simulink model "engv2_Simscape_test_no_graphs"  (R2016a)
settings: Solver=ode23t  StartTime=0.0  StopTime=5790*3  MaxStep=0.1  RelTol=1e-6
libraries: fl_lib x35, nesl_utility x35, elec_lib x10, simulink x2
settings Model: Creator=Bruno  LastModifiedBy=Bruno Eiterer
settings SolverCC: MaxConsecutiveZCs=10000  ZeroCrossAlgorithm=Adaptive  AlgebraicLoopSolver=LineSearch  SolverResetMethod=Robust

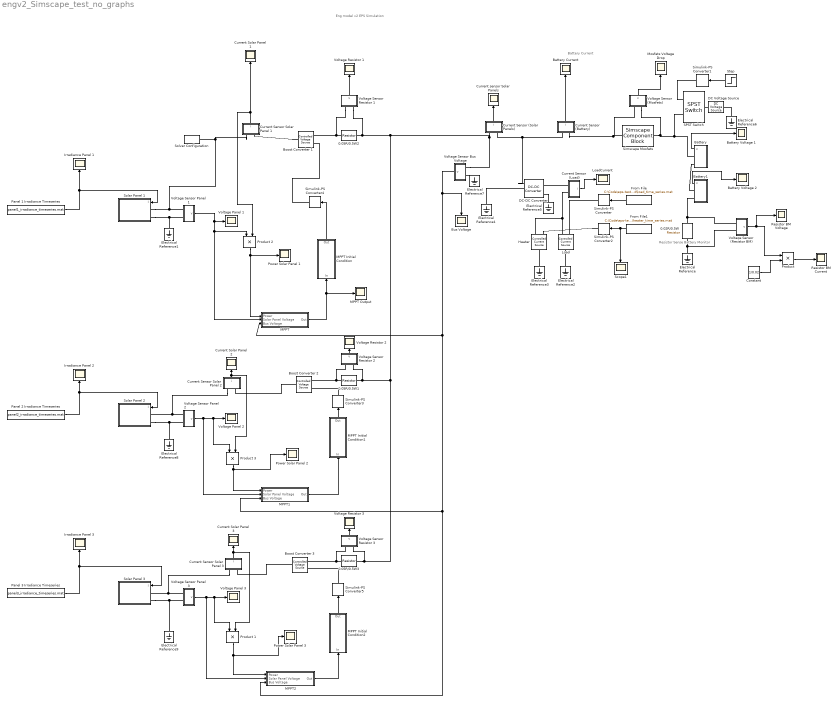
== system engv2_Simscape_test_no_graphs ==
  note: Battery Current
  note: Resistor Sense
      | Battery Monitor
  note: Eng model v2 EPS Simulation
  " Battery" : Subsystem
      settings: CopyFcn=set_param(gcb,'LinkStatus','none')
  " Battery1" : Subsystem
      settings: CopyFcn=set_param(gcb,'LinkStatus','none')
  " 0.02R/0.5W" : elec_lib/Passive Devices/Resistor  R=0.02 Ohm  R_tol=0.01  enable_R_tol=0  tol_distribution=1  nSigma=4  enable_operating_limits=0  operating_limit_action=2  max_working_voltage=100 V  power_rating=1 W  enable_faults=0  fault_action=1  R_faulted=Inf Ohm  enable_temporal_fault=0  t_fault=1 s  enable_behavioral_fault=0  max_permissible_current=1 A  t_fail_on_current=1 s  noise_mode=0  sample_time=0.001 s  repeatability=1  auto_seed=1471942077  user_seed=0  Tdevice=25 degC  alpha=0.00393 1/K  Tmeas=25 degC  thermal_mass=100 J/K  initial_temperature=25 degC  power_derating_T1=70 degC  power_derating_T2=155 degC  operating_temperature_range_vec=[ -50 150 ] degC
  " 0.05R/0.5W1" : elec_lib/Passive Devices/Resistor  R=0.02 Ohm  R_tol=0.01  enable_R_tol=0  tol_distribution=1  nSigma=4  enable_operating_limits=0  operating_limit_action=2  max_working_voltage=100 V  power_rating=1 W  enable_faults=0  fault_action=1  R_faulted=Inf Ohm  enable_temporal_fault=0  t_fault=1 s  enable_behavioral_fault=0  max_permissible_current=1 A  t_fail_on_current=1 s  noise_mode=0  sample_time=0.001 s  repeatability=1  auto_seed=2264060836  user_seed=0  Tdevice=25 degC  alpha=0.00393 1/K  Tmeas=25 degC  thermal_mass=100 J/K  initial_temperature=25 degC  power_derating_T1=70 degC  power_derating_T2=155 degC  operating_temperature_range_vec=[ -50 150 ] degC
  " 0.05R/0.5W2" : elec_lib/Passive Devices/Resistor  R=0.02 Ohm  R_tol=0.01  enable_R_tol=0  tol_distribution=1  nSigma=4  enable_operating_limits=0  operating_limit_action=2  max_working_voltage=100 V  power_rating=1 W  enable_faults=0  fault_action=1  R_faulted=Inf Ohm  enable_temporal_fault=0  t_fault=1 s  enable_behavioral_fault=0  max_permissible_current=1 A  t_fail_on_current=1 s  noise_mode=0  sample_time=0.001 s  repeatability=1  auto_seed=1206908585  user_seed=0  Tdevice=25 degC  alpha=0.00393 1/K  Tmeas=25 degC  thermal_mass=100 J/K  initial_temperature=25 degC  power_derating_T1=70 degC  power_derating_T2=155 degC  operating_temperature_range_vec=[ -50 150 ] degC
  " 0.05R/0.5W3" : elec_lib/Passive Devices/Resistor  R=0.02 Ohm  R_tol=0.01  enable_R_tol=0  tol_distribution=1  nSigma=4  enable_operating_limits=0  operating_limit_action=2  max_working_voltage=100 V  power_rating=1 W  enable_faults=0  fault_action=1  R_faulted=Inf Ohm  enable_temporal_fault=0  t_fault=1 s  enable_behavioral_fault=0  max_permissible_current=1 A  t_fail_on_current=1 s  noise_mode=0  sample_time=0.001 s  repeatability=1  auto_seed=1964622691  user_seed=0  Tdevice=25 degC  alpha=0.00393 1/K  Tmeas=25 degC  thermal_mass=100 J/K  initial_temperature=25 degC  power_derating_T1=70 degC  power_derating_T2=155 degC  operating_temperature_range_vec=[ -50 150 ] degC
  " Current Solar Panel 1" : Scope
  " Current Solar Panel 2" : Scope
  " Current Solar Panel 3" : Scope
  " Current sensor Solar Panels" : Scope
  Battery Current : Scope
  Battery Voltage 1 : Scope
  Battery Voltage 2 : Scope
  Boost Converter 1 : fl_lib/Electrical/Electrical Sources/Controlled Voltage Source
  Boost Converter 2 : fl_lib/Electrical/Electrical Sources/Controlled Voltage Source
  Boost Converter 3 : fl_lib/Electrical/Electrical Sources/Controlled Voltage Source
  Bus Voltage : Scope
  Constant : Constant  Value=1/0.02
  Current Sensor (Battery) : Subsystem
      settings: CopyFcn=set_param(gcb,'LinkStatus','none')
  Current Sensor (Load) : Subsystem
      settings: CopyFcn=set_param(gcb,'LinkStatus','none')
  Current Sensor (Solar Panels) : Subsystem
      settings: CopyFcn=set_param(gcb,'LinkStatus','none')
  Current Sensor Solar Panel 1 : Subsystem
      settings: CopyFcn=set_param(gcb,'LinkStatus','none')
  Current Sensor Solar Panel 2 : Subsystem
      settings: CopyFcn=set_param(gcb,'LinkStatus','none')
  Current Sensor Solar Panel 3 : Subsystem
      settings: CopyFcn=set_param(gcb,'LinkStatus','none')
  DC Voltage Source : fl_lib/Electrical/Electrical Sources/DC Voltage Source  v0=8.4 V
  DC-DC Converter : elec_lib/Sources/DC-DC Converter  v_ref=5 V  P_rated=10 W  droop_param=1  droop=0.0 V/A  droop_percent=2  reversible=0  efficiency=99.9999  P_fixed=0.0001 mW  model_dynamics=0  tau=0.02 s  v_ini=10 V  i1_max=10 A  fault_condition=1  fault_threshold=0.5  R_fixed=100 Ohm  R_out=0.1 Ohm  fault_sign=1
  Electrical Reference{,1..9} (10 alike) : fl_lib/Electrical/Electrical Elements/Electrical Reference
  From File : FromFile  FileName=C:\Code\eps-tests\Load\load_time_series.mat
  From File1 : FromFile  FileName=C:\Code\eps-tests\Load\heater_time_series.mat
  Heater : fl_lib/Electrical/Electrical Sources/Controlled Current Source
  Irradiance Panel 1 : Scope
  Irradiance Panel 2 : Scope
  Irradiance Panel 3 : Scope
  Load : fl_lib/Electrical/Electrical Sources/Controlled Current Source
  LoadCurrent : Scope
  MPPT : Subsystem
  MPPT Initial Condition : Subsystem
  MPPT Initial Condition1 : Subsystem
  MPPT Initial Condition2 : Subsystem
  MPPT Output : Scope
  MPPT1 : Subsystem
  MPPT2 : Subsystem
  Mosfets Voltage Drop : Scope
  Panel 1 Irradiance Timeseries : FromFile  FileName=panel1_irradiance_timeseries.mat
  Panel 2 Irradiance Timeseries : FromFile  FileName=panel2_irradiance_timeseries.mat
  Panel 3 Irradiance Timeseries : FromFile  FileName=panel3_irradiance_timeseries.mat
  Power Solar Panel 1 : Scope
  Power Solar Panel 2 : Scope
  Power Solar Panel 3 : Scope
  Product : Product
  Product 1 : Product
  "Product 2 " : Product
  Product 3 : Product
  Resistor BM Current : Scope
  Resistor BM Voltage : Scope
  SPST Switch : elec_lib/Passive Devices/Switches/SPST Switch  R_closed=0.01 Ohm  G_open=1e-6 S  Threshold=0 V  Width=0 V  model_dynamics=0  t_on=0.001 s  t_off=0.001 s  initial_vT=0 V
  Scope1 : Scope
  "Simscape Mosfets " : SimscapeComponentBlock  SourceFile=MOSFETs_EPS  ComponentPath=MOSFETs_EPS  ComponentVariants=MOSFETs_EPS  ComponentVariantNames=MOSFETs_EPS  ClassName=MOSFETs_EPS  SchemaVersion=1  Vt=1.38e-23 * 298 / 1.60e-19 V  Rsd=0.27 Ohm  Rs=0.008235 Ohm  n=1.89492  Is=1.26064e-7 A  i_specify=off  i_priority=None  i=1 A  v_specify=off  v_priority=None  v=2 V  Vr_DC_specify=off  Vr_DC_priority=None  Vr_DC=0 V  Vr_CC_specify=off  Vr_CC_priority=None  Vr_CC=0 V
      settings: CopyFcn=simscape.engine.sli.internal.componentblockcallback(gcbh,'COPY')  PreCopyFcn=simscape.engine.sli.internal.componentblockcallback(gcbh,'PRECOPY')  PreDeleteFcn=simscape.engine.sli.internal.componentblockcallback(gcbh,'PREDELETE')
      mask Type: Code produced by Embedded Systems Group - UFSC
      mask Display:
      | disp('Simscape\n\n\n')
      | disp('\n\n\nMOSFETs_EPS');
      | color('red');
      | port_label('RConn', 1,'-');
      | port_label('LConn', 1,'+');
  Simulink-PS Converter{,1..5} (6 alike) : nesl_utility/Simulink-PS Converter  PhysicalDomain=network_engine_domain  SubClassName=ps_input  LeftPortType=input  RightPortType=output  PseudoPeriodic=off  Frequencies=[]  NoiseDistribution=none  NoiseParameters=[]  Unit=1  AffineConversion=off  InputFiltering=off  SimscapeFilterOrder=1  InputFilterTimeConstant=0.001  UdotUserProvided=1
  Solar Panel 1 : Subsystem
      settings: CopyFcn=set_param(gcb,'LinkStatus','none')
  Solar Panel 2 : Subsystem
      settings: CopyFcn=set_param(gcb,'LinkStatus','none')
  Solar Panel 3 : Subsystem
      settings: CopyFcn=set_param(gcb,'LinkStatus','none')
  Solver Configuration : nesl_utility/Solver Configuration  PhysicalDomain=network_engine_domain  SubClassName=solver  LeftPortType=input  RightPortType=generic  Accelerate=off  Tones=[]  Harmonics=[]  SimulateNoise=off  Profile=off  UseLocalSampling=off  EnableSwitchedLinearOptims=on  FrequencyDomain=off  UseCCode=off  RelTol=0.001  AbsTol=1e-06  MinStep=1e-09  ToWorkspace=off  RevertToSquareIcSolve=off  NumHomotopyIterations=100  PhasorMode=off  PhasorModeNumHarmonics=1  OverrideAbsTol=off  DoDC=off  ResidualTolerance=1e-6  UseLocalSolver=off  LocalSolverChoice=NE_BACKWARD_EULER_ADVANCER  LocalSolverSampleTime=.001  DoFixedCost=off  MaxNonlinIter=3  MaxModeIter=2  LinearAlgebra=Sparse  DelaysMemoryBudget=1024  AutomaticFiltering=on  FilteringTimeConstant=0.001
  Step : Step  Before=1  After=0  SampleTime=0
  Voltage Panel 1 : Scope
  Voltage Panel 2 : Scope
  Voltage Panel 3 : Scope
  Voltage Sensor (Mosfets) : Subsystem
      settings: CopyFcn=set_param(gcb,'LinkStatus','none')
  Voltage Sensor (Resistor BM) : Subsystem
      settings: CopyFcn=set_param(gcb,'LinkStatus','none')
  Voltage Resistor 1 : Scope
  Voltage Resistor 2 : Scope
  Voltage Resistor 3 : Scope
  Voltage Sensor Bus Voltage : Subsystem
      settings: CopyFcn=set_param(gcb,'LinkStatus','none')
  Voltage Sensor Resistor 1 : Subsystem
      settings: CopyFcn=set_param(gcb,'LinkStatus','none')
  Voltage Sensor Resistor 2 : Subsystem
      settings: CopyFcn=set_param(gcb,'LinkStatus','none')
  Voltage Sensor Resistor 3 : Subsystem
      settings: CopyFcn=set_param(gcb,'LinkStatus','none')
  Voltage Sensor Panel 1 : Subsystem
      settings: CopyFcn=set_param(gcb,'LinkStatus','none')
  Voltage Sensor Panel 2 : Subsystem
      settings: CopyFcn=set_param(gcb,'LinkStatus','none')
  Voltage Sensor Panel 3 : Subsystem
      settings: CopyFcn=set_param(gcb,'LinkStatus','none')
  wires:
  Voltage Sensor (Mosfets)/1(v) -> Mosfets Voltage Drop/1
  " Battery"/1(v) -> Battery Voltage 1/1
  Current Sensor (Solar Panels)/1(i) -> " Current sensor Solar Panels"/1
  Voltage Sensor (Resistor BM)/1(v) -> Product/1, Resistor BM Voltage/1
  Current Sensor (Battery)/1(i) -> Battery Current/1
  Current Sensor Solar Panel 1/1(i) -> "Product 2 "/2, " Current Solar Panel 1"/1
  Step/1 -> Simulink-PS Converter1/1
  Current Sensor (Load)/1(i) -> LoadCurrent/1
  From File/1 -> Simulink-PS Converter/1
  From File1/1 -> Scope1/1, Simulink-PS Converter2/1
  Panel 1 Irradiance Timeseries/1 -> Solar Panel 1/1(I), Irradiance Panel 1/1
  Constant/1 -> Product/2
  Product/1 -> Resistor BM Current/1
  " Battery1"/1(v) -> Battery Voltage 2/1
  Voltage Sensor Panel 1/1(v) -> MPPT/2("Solar Panel Voltage "), "Product 2 "/1, Voltage Panel 1/1
  "Product 2 "/1 -> MPPT/1(Power), Power Solar Panel 1/1
  Voltage Sensor Bus Voltage/1(v) -> MPPT2/3(Bus Voltage), MPPT1/3(Bus Voltage), MPPT/3(Bus Voltage), Bus Voltage/1
  MPPT Initial Condition/1(Out) -> Simulink-PS Converter4/1
  MPPT/1(Out) -> MPPT Output/1, MPPT Initial Condition/1(In)
  Panel 2 Irradiance Timeseries/1 -> Irradiance Panel 2/1, Solar Panel 2/1(I)
  Voltage Sensor Panel 2/1(v) -> MPPT1/2("Solar Panel Voltage "), Product 3/1, Voltage Panel 2/1
  Product 3/1 -> MPPT1/1(Power), Power Solar Panel 2/1
  Current Sensor Solar Panel 2/1(i) -> Product 3/2, " Current Solar Panel 2"/1
  MPPT1/1(Out) -> MPPT Initial Condition1/1(In)
  MPPT Initial Condition1/1(Out) -> Simulink-PS Converter3/1
  Panel 3 Irradiance Timeseries/1 -> Irradiance Panel 3/1, Solar Panel 3/1(I)
  Current Sensor Solar Panel 3/1(i) -> Product 1/2, " Current Solar Panel 3"/1
  Voltage Sensor Panel 3/1(v) -> MPPT2/2("Solar Panel Voltage "), Product 1/1, Voltage Panel 3/1
  Product 1/1 -> MPPT2/1(Power), Power Solar Panel 3/1
  MPPT2/1(Out) -> MPPT Initial Condition2/1(In)
  MPPT Initial Condition2/1(Out) -> Simulink-PS Converter5/1
  Voltage Sensor Resistor 1/1(v) -> Voltage Resistor 1/1
  Voltage Sensor Resistor 2/1(v) -> Voltage Resistor 2/1
  Voltage Sensor Resistor 3/1(v) -> Voltage Resistor 3/1
  connections:
  Voltage Sensor (Resistor BM)/LConn1 -- " Battery1"/RConn2 -- " 0.02R/0.5W"/LConn1
  " 0.05R/0.5W2"/RConn1 -- Voltage Sensor Resistor 3/LConn2 -- " 0.05R/0.5W3"/RConn1 -- Voltage Sensor Resistor 2/LConn2 -- " 0.05R/0.5W1"/RConn1 -- Voltage Sensor Bus Voltage/LConn1 -- Current Sensor (Solar Panels)/LConn1 -- Voltage Sensor Resistor 1/LConn2
  Solver Configuration/RConn1 -- Voltage Sensor Panel 1/LConn1 -- Solar Panel 1/LConn1 -- Current Sensor Solar Panel 1/LConn1
  Current Sensor (Battery)/LConn1 -- DC-DC Converter/LConn1 -- Current Sensor (Solar Panels)/LConn2
  " 0.02R/0.5W"/RConn1 -- Electrical Reference/LConn1 -- Voltage Sensor (Resistor BM)/LConn2
  Current Sensor (Battery)/LConn2 -- "Simscape Mosfets "/LConn1 -- Voltage Sensor (Mosfets)/LConn1
  Solar Panel 1/LConn2 -- Voltage Sensor Panel 1/LConn2 -- Electrical Reference1/LConn1
  Electrical Reference2/LConn1 -- Load/LConn1
  Current Sensor (Load)/LConn2 -- Heater/RConn2 -- Load/RConn2
  Electrical Reference4/LConn1 -- DC-DC Converter/LConn2
  DC-DC Converter/RConn2 -- Electrical Reference5/LConn1
  Simulink-PS Converter1/RConn1 -- SPST Switch/LConn1
  Simulink-PS Converter/RConn1 -- Load/RConn1
  Electrical Reference6/LConn1 -- DC Voltage Source/RConn1
  Current Sensor (Load)/LConn1 -- DC-DC Converter/RConn1
  DC Voltage Source/LConn1 -- SPST Switch/RConn1
  Electrical Reference3/LConn1 -- Heater/LConn1
  Simulink-PS Converter2/RConn1 -- Heater/RConn1
  " Battery1"/RConn1 -- " Battery"/RConn2
  Voltage Sensor Bus Voltage/LConn2 -- Electrical Reference7/LConn1
  Simulink-PS Converter4/RConn1 -- Boost Converter 1/RConn1
  SPST Switch/LConn2 -- "Simscape Mosfets "/RConn1 -- Voltage Sensor (Mosfets)/LConn2 -- " Battery"/RConn1
  Boost Converter 1/LConn1 -- Current Sensor Solar Panel 1/LConn2
  Voltage Sensor Panel 2/LConn1 -- Solar Panel 2/LConn1 -- Current Sensor Solar Panel 2/LConn1
  Solar Panel 2/LConn2 -- Electrical Reference8/LConn1 -- Voltage Sensor Panel 2/LConn2
  Boost Converter 2/LConn1 -- Current Sensor Solar Panel 2/LConn2
  Simulink-PS Converter3/RConn1 -- Boost Converter 2/RConn1
  Voltage Sensor Panel 3/LConn1 -- Current Sensor Solar Panel 3/LConn1 -- Solar Panel 3/LConn1
  Solar Panel 3/LConn2 -- Electrical Reference9/LConn1 -- Voltage Sensor Panel 3/LConn2
  Boost Converter 3/LConn1 -- Current Sensor Solar Panel 3/LConn2
  Simulink-PS Converter5/RConn1 -- Boost Converter 3/RConn1
  " 0.05R/0.5W2"/LConn1 -- Boost Converter 1/RConn2 -- Voltage Sensor Resistor 1/LConn1
  " 0.05R/0.5W1"/LConn1 -- Boost Converter 2/RConn2 -- Voltage Sensor Resistor 2/LConn1
  " 0.05R/0.5W3"/LConn1 -- Voltage Sensor Resistor 3/LConn1 -- Boost Converter 3/RConn2

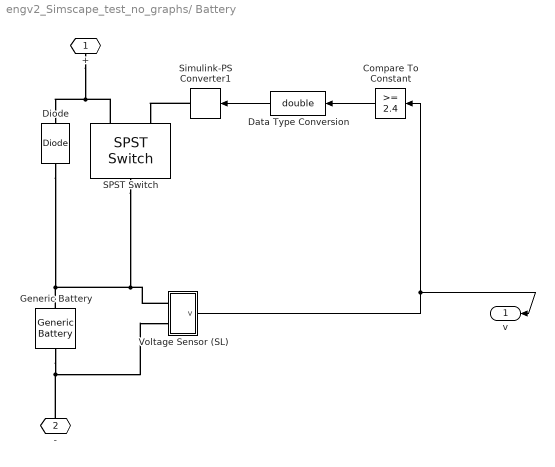
== system engv2_Simscape_test_no_graphs/ Battery ==
  Compare To Constant : simulink/Logic and Bit Operations/Compare To Constant  relop=>=  const=2.4  OutDataTypeStr=boolean
  Data Type Conversion : DataTypeConversion  OutDataTypeStr=double
  Diode : fl_lib/Electrical/Electrical Elements/Diode  Vf=0.0001 V  Ron=0.0001 Ohm  Goff=1e-8 1/Ohm  i_specify=off  i_priority=None  i=0 A  v_specify=off  v_priority=None  v=0 V
  Generic Battery : elec_lib/Sources/Generic Battery  Vnom=4.1 V  R1=0.01 Ohm  prm_AH=2  AH=3 hr*A  AH0=3 hr*A  V1=3.789 V  AH1=2.19 hr*A  prm_R2=1  R2=2e+3 Ohm
  SPST Switch : elec_lib/Passive Devices/Switches/SPST Switch  R_closed=0.01 Ohm  G_open=1e-6 S  Threshold=0 V  Width=0.1 V  model_dynamics=0  t_on=0.001 s  t_off=0.001 s  initial_vT=0 V
  Simulink-PS Converter1 : nesl_utility/Simulink-PS Converter  PhysicalDomain=network_engine_domain  SubClassName=ps_input  LeftPortType=input  RightPortType=output  PseudoPeriodic=off  Frequencies=[]  NoiseDistribution=none  NoiseParameters=[]  Unit=V  AffineConversion=off  InputFiltering=off  SimscapeFilterOrder=1  InputFilterTimeConstant=.001  UdotUserProvided=1
  Voltage Sensor (SL) : Subsystem
      settings: CopyFcn=set_param(gcb,'LinkStatus','none')
  + : PMIOPort  Port=1  Side=Right
  - : PMIOPort  Port=2  Side=Right
  v : Outport
  wires:
  Voltage Sensor (SL)/1(v) -> v/1, Compare To Constant/1
  Data Type Conversion/1 -> Simulink-PS Converter1/1
  Compare To Constant/1 -> Data Type Conversion/1
  connections:
  -/RConn1 -- Generic Battery/RConn1 -- Voltage Sensor (SL)/LConn2
  Voltage Sensor (SL)/LConn1 -- SPST Switch/RConn1 -- Diode/RConn1 -- Generic Battery/LConn1
  +/RConn1 -- Diode/LConn1 -- SPST Switch/LConn2
  Simulink-PS Converter1/RConn1 -- SPST Switch/LConn1

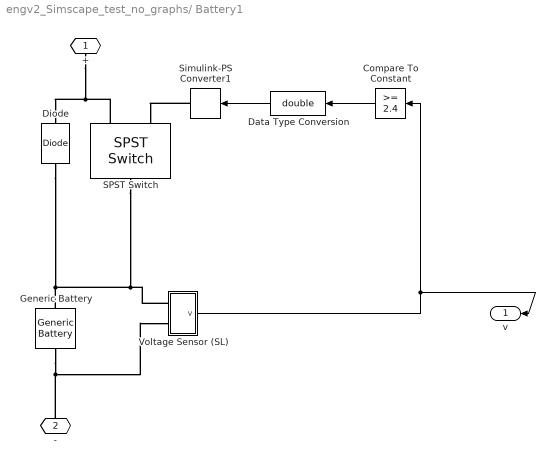
== system engv2_Simscape_test_no_graphs/ Battery1 ==
  Compare To Constant : simulink/Logic and Bit Operations/Compare To Constant  relop=>=  const=2.4  OutDataTypeStr=boolean
  Data Type Conversion : DataTypeConversion  OutDataTypeStr=double
  Diode : fl_lib/Electrical/Electrical Elements/Diode  Vf=0.0001 V  Ron=0.0001 Ohm  Goff=1e-8 1/Ohm  i_specify=off  i_priority=None  i=0 A  v_specify=off  v_priority=None  v=0 V
  Generic Battery : elec_lib/Sources/Generic Battery  Vnom=4.1 V  R1=0.01 Ohm  prm_AH=2  AH=3 hr*A  AH0=3 hr*A  V1=3.789 V  AH1=2.19 hr*A  prm_R2=1  R2=2e+3 Ohm
  SPST Switch : elec_lib/Passive Devices/Switches/SPST Switch  R_closed=0.01 Ohm  G_open=1e-6 S  Threshold=0 V  Width=0.1 V  model_dynamics=0  t_on=0.001 s  t_off=0.001 s  initial_vT=0 V
  Simulink-PS Converter1 : nesl_utility/Simulink-PS Converter  PhysicalDomain=network_engine_domain  SubClassName=ps_input  LeftPortType=input  RightPortType=output  PseudoPeriodic=off  Frequencies=[]  NoiseDistribution=none  NoiseParameters=[]  Unit=V  AffineConversion=off  InputFiltering=off  SimscapeFilterOrder=1  InputFilterTimeConstant=.001  UdotUserProvided=1
  Voltage Sensor (SL) : Subsystem
      settings: CopyFcn=set_param(gcb,'LinkStatus','none')
  + : PMIOPort  Port=1  Side=Right
  - : PMIOPort  Port=2  Side=Right
  v : Outport
  wires:
  Voltage Sensor (SL)/1(v) -> v/1, Compare To Constant/1
  Data Type Conversion/1 -> Simulink-PS Converter1/1
  Compare To Constant/1 -> Data Type Conversion/1
  connections:
  -/RConn1 -- Generic Battery/RConn1 -- Voltage Sensor (SL)/LConn2
  Voltage Sensor (SL)/LConn1 -- SPST Switch/RConn1 -- Diode/RConn1 -- Generic Battery/LConn1
  +/RConn1 -- Diode/LConn1 -- SPST Switch/LConn2
  Simulink-PS Converter1/RConn1 -- SPST Switch/LConn1

== system engv2_Simscape_test_no_graphs/Current Sensor (Battery) ==
  Current Sensor : fl_lib/Electrical/Electrical Sensors/Current Sensor
  PS-Simulink : nesl_utility/PS-Simulink Converter  PhysicalDomain=network_engine_domain  SubClassName=ps_output  LeftPortType=input  RightPortType=output  PseudoPeriodic=off  Frequencies=[]  Unit=A  AffineConversion=off
  + : PMIOPort  Port=1  Side=Left
  - : PMIOPort  Port=2  Side=Left
  i : Outport
  wires:
  PS-Simulink/1 -> i/1
  connections:
  -/RConn1 -- Current Sensor/RConn2
  +/RConn1 -- Current Sensor/LConn1
  Current Sensor/RConn1 -- PS-Simulink/LConn1

== system engv2_Simscape_test_no_graphs/Current Sensor (Load) ==
  Current Sensor : fl_lib/Electrical/Electrical Sensors/Current Sensor
  PS-Simulink : nesl_utility/PS-Simulink Converter  PhysicalDomain=network_engine_domain  SubClassName=ps_output  LeftPortType=input  RightPortType=output  PseudoPeriodic=off  Frequencies=[]  Unit=A  AffineConversion=off
  + : PMIOPort  Port=1  Side=Left
  - : PMIOPort  Port=2  Side=Left
  i : Outport
  wires:
  PS-Simulink/1 -> i/1
  connections:
  -/RConn1 -- Current Sensor/RConn2
  +/RConn1 -- Current Sensor/LConn1
  Current Sensor/RConn1 -- PS-Simulink/LConn1

== system engv2_Simscape_test_no_graphs/Current Sensor (Solar Panels) ==
  Current Sensor : fl_lib/Electrical/Electrical Sensors/Current Sensor
  PS-Simulink : nesl_utility/PS-Simulink Converter  PhysicalDomain=network_engine_domain  SubClassName=ps_output  LeftPortType=input  RightPortType=output  PseudoPeriodic=off  Frequencies=[]  Unit=A  AffineConversion=off
  + : PMIOPort  Port=1  Side=Left
  - : PMIOPort  Port=2  Side=Left
  i : Outport
  wires:
  PS-Simulink/1 -> i/1
  connections:
  -/RConn1 -- Current Sensor/RConn2
  +/RConn1 -- Current Sensor/LConn1
  Current Sensor/RConn1 -- PS-Simulink/LConn1

== system engv2_Simscape_test_no_graphs/Current Sensor Solar Panel 1 ==
  Current Sensor : fl_lib/Electrical/Electrical Sensors/Current Sensor
  PS-Simulink : nesl_utility/PS-Simulink Converter  PhysicalDomain=network_engine_domain  SubClassName=ps_output  LeftPortType=input  RightPortType=output  PseudoPeriodic=off  Frequencies=[]  Unit=A  AffineConversion=off
  + : PMIOPort  Port=1  Side=Left
  - : PMIOPort  Port=2  Side=Left
  i : Outport
  wires:
  PS-Simulink/1 -> i/1
  connections:
  -/RConn1 -- Current Sensor/RConn2
  +/RConn1 -- Current Sensor/LConn1
  Current Sensor/RConn1 -- PS-Simulink/LConn1

== system engv2_Simscape_test_no_graphs/Current Sensor Solar Panel 2 ==
  Current Sensor : fl_lib/Electrical/Electrical Sensors/Current Sensor
  PS-Simulink : nesl_utility/PS-Simulink Converter  PhysicalDomain=network_engine_domain  SubClassName=ps_output  LeftPortType=input  RightPortType=output  PseudoPeriodic=off  Frequencies=[]  Unit=A  AffineConversion=off
  + : PMIOPort  Port=1  Side=Left
  - : PMIOPort  Port=2  Side=Left
  i : Outport
  wires:
  PS-Simulink/1 -> i/1
  connections:
  -/RConn1 -- Current Sensor/RConn2
  +/RConn1 -- Current Sensor/LConn1
  Current Sensor/RConn1 -- PS-Simulink/LConn1

== system engv2_Simscape_test_no_graphs/Current Sensor Solar Panel 3 ==
  Current Sensor : fl_lib/Electrical/Electrical Sensors/Current Sensor
  PS-Simulink : nesl_utility/PS-Simulink Converter  PhysicalDomain=network_engine_domain  SubClassName=ps_output  LeftPortType=input  RightPortType=output  PseudoPeriodic=off  Frequencies=[]  Unit=A  AffineConversion=off
  + : PMIOPort  Port=1  Side=Left
  - : PMIOPort  Port=2  Side=Left
  i : Outport
  wires:
  PS-Simulink/1 -> i/1
  connections:
  -/RConn1 -- Current Sensor/RConn2
  +/RConn1 -- Current Sensor/LConn1
  Current Sensor/RConn1 -- PS-Simulink/LConn1

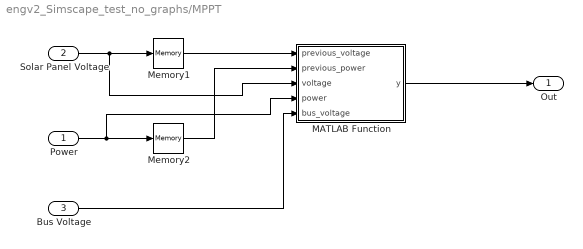
== system engv2_Simscape_test_no_graphs/MPPT ==
  Power : Inport
  "Solar Panel Voltage " : Inport  Port=2
  Bus Voltage : Inport  Port=3
  MATLAB Function : MATLAB Function  TreatAsAtomicUnit=on  SystemSampleTime=0.1
      settings: MinAlgLoopOccurrences=on
  Memory1 : Memory  X0=0.311*2.363
  Memory2 : Memory  X0=0.311*2.363
  Out : Outport
  wires:
  MATLAB Function/1(y) -> Out/1
  Memory1/1 -> MATLAB Function/1(previous_voltage)
  "Solar Panel Voltage "/1 -> MATLAB Function/3(voltage), Memory1/1
  Memory2/1 -> MATLAB Function/2(previous_power)
  Power/1 -> MATLAB Function/4(power), Memory2/1
  Bus Voltage/1 -> MATLAB Function/5(bus_voltage)

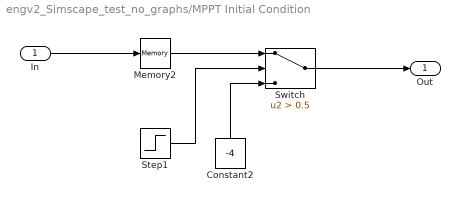
== system engv2_Simscape_test_no_graphs/MPPT Initial Condition ==
  In : Inport
  Constant2 : Constant  Value=-4
  Memory2 : Memory  X0=0.311*2.363
  Step1 : Step  SampleTime=0
  Switch : Switch  Criteria=u2 > Threshold  Threshold=0.5
  Out : Outport
  wires:
  In/1 -> Memory2/1
  Memory2/1 -> Switch/1
  Step1/1 -> Switch/2
  Constant2/1 -> Switch/3
  Switch/1 -> Out/1

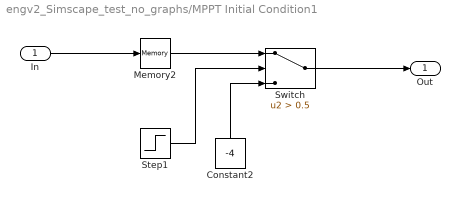
== system engv2_Simscape_test_no_graphs/MPPT Initial Condition1 ==
  In : Inport
  Constant2 : Constant  Value=-4
  Memory2 : Memory  X0=0.311*2.363
  Step1 : Step  SampleTime=0
  Switch : Switch  Criteria=u2 > Threshold  Threshold=0.5
  Out : Outport
  wires:
  In/1 -> Memory2/1
  Memory2/1 -> Switch/1
  Step1/1 -> Switch/2
  Constant2/1 -> Switch/3
  Switch/1 -> Out/1

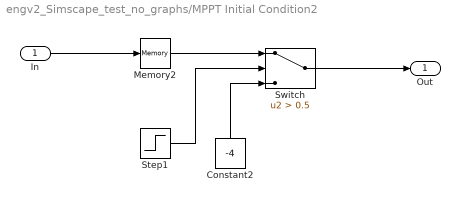
== system engv2_Simscape_test_no_graphs/MPPT Initial Condition2 ==
  In : Inport
  Constant2 : Constant  Value=-4
  Memory2 : Memory  X0=0.311*2.363
  Step1 : Step  SampleTime=0
  Switch : Switch  Criteria=u2 > Threshold  Threshold=0.5
  Out : Outport
  wires:
  In/1 -> Memory2/1
  Memory2/1 -> Switch/1
  Step1/1 -> Switch/2
  Constant2/1 -> Switch/3
  Switch/1 -> Out/1

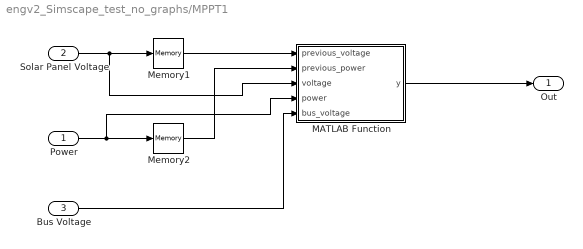
== system engv2_Simscape_test_no_graphs/MPPT1 ==
  Power : Inport
  "Solar Panel Voltage " : Inport  Port=2
  Bus Voltage : Inport  Port=3
  MATLAB Function : MATLAB Function  TreatAsAtomicUnit=on  SystemSampleTime=0.1
      settings: MinAlgLoopOccurrences=on
  Memory1 : Memory  X0=0.311*2.363
  Memory2 : Memory  X0=0.311*2.363
  Out : Outport
  wires:
  MATLAB Function/1(y) -> Out/1
  Memory1/1 -> MATLAB Function/1(previous_voltage)
  "Solar Panel Voltage "/1 -> MATLAB Function/3(voltage), Memory1/1
  Memory2/1 -> MATLAB Function/2(previous_power)
  Power/1 -> MATLAB Function/4(power), Memory2/1
  Bus Voltage/1 -> MATLAB Function/5(bus_voltage)

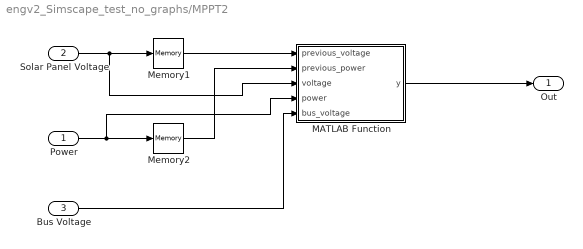
== system engv2_Simscape_test_no_graphs/MPPT2 ==
  Power : Inport
  "Solar Panel Voltage " : Inport  Port=2
  Bus Voltage : Inport  Port=3
  MATLAB Function : MATLAB Function  TreatAsAtomicUnit=on  SystemSampleTime=0.1
      settings: MinAlgLoopOccurrences=on
  Memory1 : Memory  X0=0.311*2.363
  Memory2 : Memory  X0=0.311*2.363
  Out : Outport
  wires:
  MATLAB Function/1(y) -> Out/1
  Memory1/1 -> MATLAB Function/1(previous_voltage)
  "Solar Panel Voltage "/1 -> MATLAB Function/3(voltage), Memory1/1
  Memory2/1 -> MATLAB Function/2(previous_power)
  Power/1 -> MATLAB Function/4(power), Memory2/1
  Bus Voltage/1 -> MATLAB Function/5(bus_voltage)

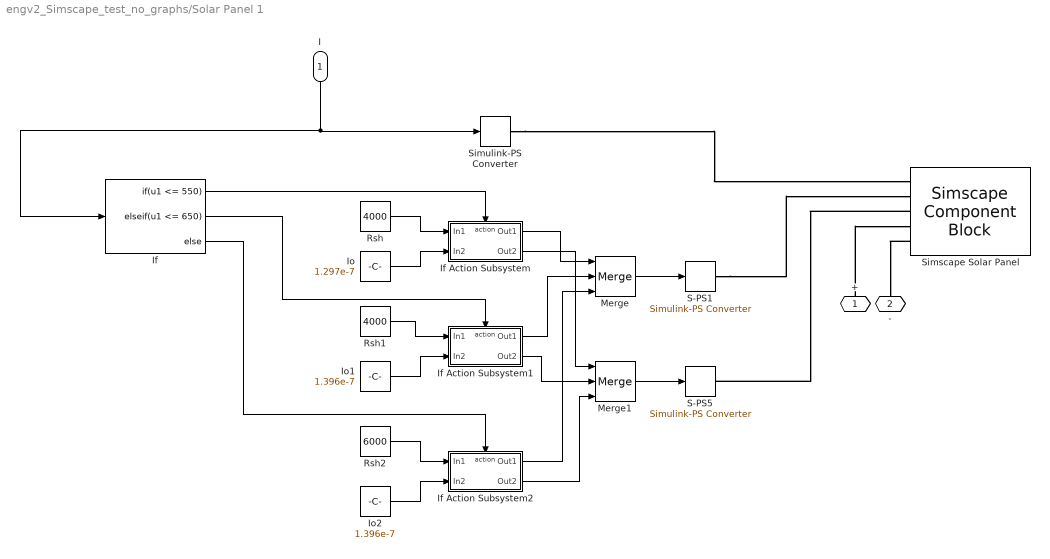
== system engv2_Simscape_test_no_graphs/Solar Panel 1 ==
  I : Inport
  If : If  IfExpression=u1 <= 550  ElseIfExpressions=u1 <= 650
  If Action Subsystem : Subsystem  TreatAsAtomicUnit=on
  If Action Subsystem1 : Subsystem  TreatAsAtomicUnit=on
  If Action Subsystem2 : Subsystem  TreatAsAtomicUnit=on
  Io : Constant  Value=1.297e-7
  Io1 : Constant  Value=1.396e-7
  Io2 : Constant  Value=1.396e-7
  Merge : Merge  Inputs=3
  Merge1 : Merge  Inputs=3
  Rsh : Constant  Value=4000
  Rsh1 : Constant  Value=4000
  Rsh2 : Constant  Value=6000
  S-PS1 : nesl_utility/Simulink-PS Converter  PhysicalDomain=network_engine_domain  SubClassName=ps_input  LeftPortType=input  RightPortType=output  PseudoPeriodic=off  Frequencies=[]  NoiseDistribution=none  NoiseParameters=[]  Unit=1  AffineConversion=off  InputFiltering=off  SimscapeFilterOrder=1  InputFilterTimeConstant=0.001  UdotUserProvided=1
  S-PS5 : nesl_utility/Simulink-PS Converter  PhysicalDomain=network_engine_domain  SubClassName=ps_input  LeftPortType=input  RightPortType=output  PseudoPeriodic=off  Frequencies=[]  NoiseDistribution=none  NoiseParameters=[]  Unit=1  AffineConversion=off  InputFiltering=off  SimscapeFilterOrder=1  InputFilterTimeConstant=0.001  UdotUserProvided=1
  Simscape Solar Panel : SimscapeComponentBlock  SourceFile=simscape.solarPanel  ComponentPath=simscape.solarPanel  ComponentVariants=simscape.solarPanel  ComponentVariantNames=solarPanel  ClassName=solarPanel  SchemaVersion=1  Rs=1 Ohm  A=2  Iph0=0.050 A  Np=4  Ns=10  Npp=1  efficiency=0.91  i_specify=off  i_priority=None  i=0 A  v_specify=off  v_priority=None  v=0 V
      settings: CopyFcn=simscape.engine.sli.internal.componentblockcallback(gcbh,'COPY')  PreCopyFcn=simscape.engine.sli.internal.componentblockcallback(gcbh,'PRECOPY')  PreDeleteFcn=simscape.engine.sli.internal.componentblockcallback(gcbh,'PREDELETE')
      mask Type: solarPanel
      mask Display:
      | disp('Simscape\n\n\n')
      | disp('\n\n\nsolarPanel');
      | color('red');
      | port_label('LConn', 5,'n');
      | port_label('LConn', 4,'p');
      | port_label('LConn', 3,'diode saturation current');
      | port_label('LConn', 2,'parallel resistance');
      | port_label('LConn', 1,'I');
  Simulink-PS Converter : nesl_utility/Simulink-PS Converter  PhysicalDomain=network_engine_domain  SubClassName=ps_input  LeftPortType=input  RightPortType=output  PseudoPeriodic=off  Frequencies=[]  NoiseDistribution=none  NoiseParameters=[]  Unit=1  AffineConversion=off  InputFiltering=off  SimscapeFilterOrder=1  InputFilterTimeConstant=0.001  UdotUserProvided=1
  + : PMIOPort  Port=1  Side=Left
  - : PMIOPort  Port=2  Side=Left
  wires:
  I/1 -> Simulink-PS Converter/1, If/1
  If/1 -> If Action Subsystem/Action
  Rsh/1 -> If Action Subsystem/1(In1)
  Io/1 -> If Action Subsystem/2(In2)
  If/2 -> If Action Subsystem1/Action
  Io1/1 -> If Action Subsystem1/2(In2)
  Rsh1/1 -> If Action Subsystem1/1(In1)
  If Action Subsystem1/1(Out1) -> Merge/2
  If Action Subsystem/1(Out1) -> Merge/1
  Merge/1 -> S-PS1/1
  If/3 -> If Action Subsystem2/Action
  Rsh2/1 -> If Action Subsystem2/1(In1)
  Io2/1 -> If Action Subsystem2/2(In2)
  If Action Subsystem2/1(Out1) -> Merge/3
  If Action Subsystem/2(Out2) -> Merge1/1
  If Action Subsystem1/2(Out2) -> Merge1/2
  If Action Subsystem2/2(Out2) -> Merge1/3
  Merge1/1 -> S-PS5/1
  connections:
  +/RConn1 -- Simscape Solar Panel/LConn4
  Simscape Solar Panel/LConn5 -- -/RConn1
  S-PS1/RConn1 -- Simscape Solar Panel/LConn2
  Simscape Solar Panel/LConn3 -- S-PS5/RConn1
  Simulink-PS Converter/RConn1 -- Simscape Solar Panel/LConn1

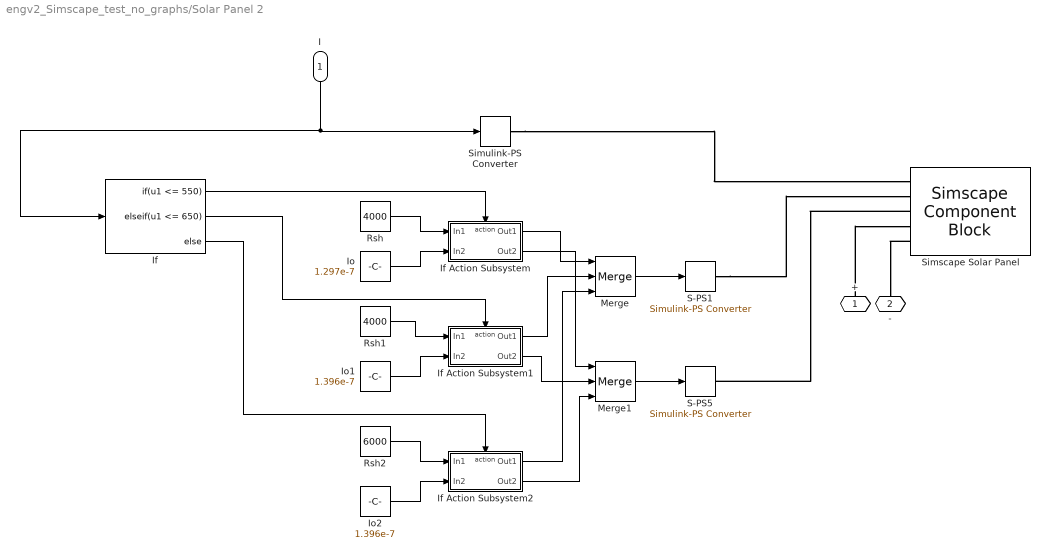
== system engv2_Simscape_test_no_graphs/Solar Panel 2 ==
  I : Inport
  If : If  IfExpression=u1 <= 550  ElseIfExpressions=u1 <= 650
  If Action Subsystem : Subsystem  TreatAsAtomicUnit=on
  If Action Subsystem1 : Subsystem  TreatAsAtomicUnit=on
  If Action Subsystem2 : Subsystem  TreatAsAtomicUnit=on
  Io : Constant  Value=1.297e-7
  Io1 : Constant  Value=1.396e-7
  Io2 : Constant  Value=1.396e-7
  Merge : Merge  Inputs=3
  Merge1 : Merge  Inputs=3
  Rsh : Constant  Value=4000
  Rsh1 : Constant  Value=4000
  Rsh2 : Constant  Value=6000
  S-PS1 : nesl_utility/Simulink-PS Converter  PhysicalDomain=network_engine_domain  SubClassName=ps_input  LeftPortType=input  RightPortType=output  PseudoPeriodic=off  Frequencies=[]  NoiseDistribution=none  NoiseParameters=[]  Unit=1  AffineConversion=off  InputFiltering=off  SimscapeFilterOrder=1  InputFilterTimeConstant=0.001  UdotUserProvided=1
  S-PS5 : nesl_utility/Simulink-PS Converter  PhysicalDomain=network_engine_domain  SubClassName=ps_input  LeftPortType=input  RightPortType=output  PseudoPeriodic=off  Frequencies=[]  NoiseDistribution=none  NoiseParameters=[]  Unit=1  AffineConversion=off  InputFiltering=off  SimscapeFilterOrder=1  InputFilterTimeConstant=0.001  UdotUserProvided=1
  Simscape Solar Panel : SimscapeComponentBlock  SourceFile=simscape.solarPanel  ComponentPath=simscape.solarPanel  ComponentVariants=simscape.solarPanel  ComponentVariantNames=solarPanel  ClassName=solarPanel  SchemaVersion=1  Rs=1 Ohm  A=2  Iph0=0.050 A  Np=4  Ns=10  Npp=1  efficiency=0.91  i_specify=off  i_priority=None  i=0 A  v_specify=off  v_priority=None  v=0 V
      settings: CopyFcn=simscape.engine.sli.internal.componentblockcallback(gcbh,'COPY')  PreCopyFcn=simscape.engine.sli.internal.componentblockcallback(gcbh,'PRECOPY')  PreDeleteFcn=simscape.engine.sli.internal.componentblockcallback(gcbh,'PREDELETE')
      mask Type: solarPanel
      mask Display:
      | disp('Simscape\n\n\n')
      | disp('\n\n\nsolarPanel');
      | color('red');
      | port_label('LConn', 5,'n');
      | port_label('LConn', 4,'p');
      | port_label('LConn', 3,'diode saturation current');
      | port_label('LConn', 2,'parallel resistance');
      | port_label('LConn', 1,'I');
  Simulink-PS Converter : nesl_utility/Simulink-PS Converter  PhysicalDomain=network_engine_domain  SubClassName=ps_input  LeftPortType=input  RightPortType=output  PseudoPeriodic=off  Frequencies=[]  NoiseDistribution=none  NoiseParameters=[]  Unit=1  AffineConversion=off  InputFiltering=off  SimscapeFilterOrder=1  InputFilterTimeConstant=0.001  UdotUserProvided=1
  + : PMIOPort  Port=1  Side=Left
  - : PMIOPort  Port=2  Side=Left
  wires:
  I/1 -> Simulink-PS Converter/1, If/1
  If/1 -> If Action Subsystem/Action
  Rsh/1 -> If Action Subsystem/1(In1)
  Io/1 -> If Action Subsystem/2(In2)
  If/2 -> If Action Subsystem1/Action
  Io1/1 -> If Action Subsystem1/2(In2)
  Rsh1/1 -> If Action Subsystem1/1(In1)
  If Action Subsystem1/1(Out1) -> Merge/2
  If Action Subsystem/1(Out1) -> Merge/1
  Merge/1 -> S-PS1/1
  If/3 -> If Action Subsystem2/Action
  Rsh2/1 -> If Action Subsystem2/1(In1)
  Io2/1 -> If Action Subsystem2/2(In2)
  If Action Subsystem2/1(Out1) -> Merge/3
  If Action Subsystem/2(Out2) -> Merge1/1
  If Action Subsystem1/2(Out2) -> Merge1/2
  If Action Subsystem2/2(Out2) -> Merge1/3
  Merge1/1 -> S-PS5/1
  connections:
  +/RConn1 -- Simscape Solar Panel/LConn4
  Simscape Solar Panel/LConn5 -- -/RConn1
  S-PS1/RConn1 -- Simscape Solar Panel/LConn2
  Simscape Solar Panel/LConn3 -- S-PS5/RConn1
  Simulink-PS Converter/RConn1 -- Simscape Solar Panel/LConn1

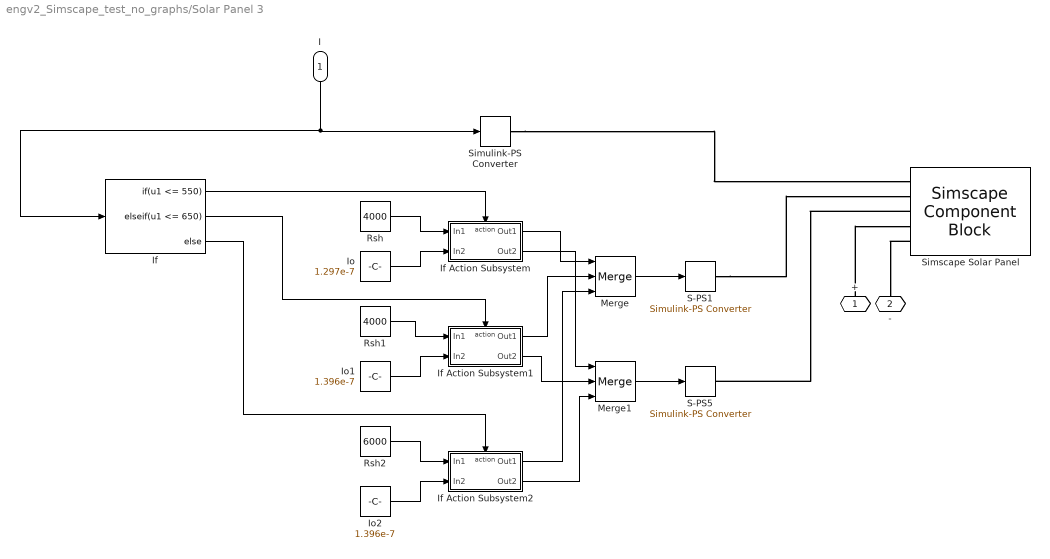
== system engv2_Simscape_test_no_graphs/Solar Panel 3 ==
  I : Inport
  If : If  IfExpression=u1 <= 550  ElseIfExpressions=u1 <= 650
  If Action Subsystem : Subsystem  TreatAsAtomicUnit=on
  If Action Subsystem1 : Subsystem  TreatAsAtomicUnit=on
  If Action Subsystem2 : Subsystem  TreatAsAtomicUnit=on
  Io : Constant  Value=1.297e-7
  Io1 : Constant  Value=1.396e-7
  Io2 : Constant  Value=1.396e-7
  Merge : Merge  Inputs=3
  Merge1 : Merge  Inputs=3
  Rsh : Constant  Value=4000
  Rsh1 : Constant  Value=4000
  Rsh2 : Constant  Value=6000
  S-PS1 : nesl_utility/Simulink-PS Converter  PhysicalDomain=network_engine_domain  SubClassName=ps_input  LeftPortType=input  RightPortType=output  PseudoPeriodic=off  Frequencies=[]  NoiseDistribution=none  NoiseParameters=[]  Unit=1  AffineConversion=off  InputFiltering=off  SimscapeFilterOrder=1  InputFilterTimeConstant=0.001  UdotUserProvided=1
  S-PS5 : nesl_utility/Simulink-PS Converter  PhysicalDomain=network_engine_domain  SubClassName=ps_input  LeftPortType=input  RightPortType=output  PseudoPeriodic=off  Frequencies=[]  NoiseDistribution=none  NoiseParameters=[]  Unit=1  AffineConversion=off  InputFiltering=off  SimscapeFilterOrder=1  InputFilterTimeConstant=0.001  UdotUserProvided=1
  Simscape Solar Panel : SimscapeComponentBlock  SourceFile=simscape.solarPanel  ComponentPath=simscape.solarPanel  ComponentVariants=simscape.solarPanel  ComponentVariantNames=solarPanel  ClassName=solarPanel  SchemaVersion=1  Rs=1 Ohm  A=2  Iph0=0.050 A  Np=4  Ns=10  Npp=1  efficiency=0.91  i_specify=off  i_priority=None  i=0 A  v_specify=off  v_priority=None  v=0 V
      settings: CopyFcn=simscape.engine.sli.internal.componentblockcallback(gcbh,'COPY')  PreCopyFcn=simscape.engine.sli.internal.componentblockcallback(gcbh,'PRECOPY')  PreDeleteFcn=simscape.engine.sli.internal.componentblockcallback(gcbh,'PREDELETE')
      mask Type: solarPanel
      mask Display:
      | disp('Simscape\n\n\n')
      | disp('\n\n\nsolarPanel');
      | color('red');
      | port_label('LConn', 5,'n');
      | port_label('LConn', 4,'p');
      | port_label('LConn', 3,'diode saturation current');
      | port_label('LConn', 2,'parallel resistance');
      | port_label('LConn', 1,'I');
  Simulink-PS Converter : nesl_utility/Simulink-PS Converter  PhysicalDomain=network_engine_domain  SubClassName=ps_input  LeftPortType=input  RightPortType=output  PseudoPeriodic=off  Frequencies=[]  NoiseDistribution=none  NoiseParameters=[]  Unit=1  AffineConversion=off  InputFiltering=off  SimscapeFilterOrder=1  InputFilterTimeConstant=0.001  UdotUserProvided=1
  + : PMIOPort  Port=1  Side=Left
  - : PMIOPort  Port=2  Side=Left
  wires:
  I/1 -> Simulink-PS Converter/1, If/1
  If/1 -> If Action Subsystem/Action
  Rsh/1 -> If Action Subsystem/1(In1)
  Io/1 -> If Action Subsystem/2(In2)
  If/2 -> If Action Subsystem1/Action
  Io1/1 -> If Action Subsystem1/2(In2)
  Rsh1/1 -> If Action Subsystem1/1(In1)
  If Action Subsystem1/1(Out1) -> Merge/2
  If Action Subsystem/1(Out1) -> Merge/1
  Merge/1 -> S-PS1/1
  If/3 -> If Action Subsystem2/Action
  Rsh2/1 -> If Action Subsystem2/1(In1)
  Io2/1 -> If Action Subsystem2/2(In2)
  If Action Subsystem2/1(Out1) -> Merge/3
  If Action Subsystem/2(Out2) -> Merge1/1
  If Action Subsystem1/2(Out2) -> Merge1/2
  If Action Subsystem2/2(Out2) -> Merge1/3
  Merge1/1 -> S-PS5/1
  connections:
  +/RConn1 -- Simscape Solar Panel/LConn4
  Simscape Solar Panel/LConn5 -- -/RConn1
  S-PS1/RConn1 -- Simscape Solar Panel/LConn2
  Simscape Solar Panel/LConn3 -- S-PS5/RConn1
  Simulink-PS Converter/RConn1 -- Simscape Solar Panel/LConn1

== system engv2_Simscape_test_no_graphs/Voltage Sensor (Mosfets) ==
  PS-Simulink : nesl_utility/PS-Simulink Converter  PhysicalDomain=network_engine_domain  SubClassName=ps_output  LeftPortType=input  RightPortType=output  PseudoPeriodic=off  Frequencies=[]  Unit=V  AffineConversion=off
  Voltage Sensor : fl_lib/Electrical/Electrical Sensors/Voltage Sensor
  + : PMIOPort  Port=1  Side=Left
  - : PMIOPort  Port=2  Side=Left
  v : Outport
  wires:
  PS-Simulink/1 -> v/1
  connections:
  -/RConn1 -- Voltage Sensor/RConn2
  +/RConn1 -- Voltage Sensor/LConn1
  Voltage Sensor/RConn1 -- PS-Simulink/LConn1

== system engv2_Simscape_test_no_graphs/Voltage Sensor (Resistor BM) ==
  PS-Simulink : nesl_utility/PS-Simulink Converter  PhysicalDomain=network_engine_domain  SubClassName=ps_output  LeftPortType=input  RightPortType=output  PseudoPeriodic=off  Frequencies=[]  Unit=V  AffineConversion=off
  Voltage Sensor : fl_lib/Electrical/Electrical Sensors/Voltage Sensor
  + : PMIOPort  Port=1  Side=Left
  - : PMIOPort  Port=2  Side=Left
  v : Outport
  wires:
  PS-Simulink/1 -> v/1
  connections:
  -/RConn1 -- Voltage Sensor/RConn2
  +/RConn1 -- Voltage Sensor/LConn1
  Voltage Sensor/RConn1 -- PS-Simulink/LConn1

== system engv2_Simscape_test_no_graphs/Voltage Sensor Bus Voltage ==
  PS-Simulink : nesl_utility/PS-Simulink Converter  PhysicalDomain=network_engine_domain  SubClassName=ps_output  LeftPortType=input  RightPortType=output  PseudoPeriodic=off  Frequencies=[]  Unit=V  AffineConversion=off
  Voltage Sensor : fl_lib/Electrical/Electrical Sensors/Voltage Sensor
  + : PMIOPort  Port=1  Side=Left
  - : PMIOPort  Port=2  Side=Left
  v : Outport
  wires:
  PS-Simulink/1 -> v/1
  connections:
  -/RConn1 -- Voltage Sensor/RConn2
  +/RConn1 -- Voltage Sensor/LConn1
  Voltage Sensor/RConn1 -- PS-Simulink/LConn1

== system engv2_Simscape_test_no_graphs/Voltage Sensor Resistor 1 ==
  PS-Simulink : nesl_utility/PS-Simulink Converter  PhysicalDomain=network_engine_domain  SubClassName=ps_output  LeftPortType=input  RightPortType=output  PseudoPeriodic=off  Frequencies=[]  Unit=V  AffineConversion=off
  Voltage Sensor : fl_lib/Electrical/Electrical Sensors/Voltage Sensor
  + : PMIOPort  Port=1  Side=Left
  - : PMIOPort  Port=2  Side=Left
  v : Outport
  wires:
  PS-Simulink/1 -> v/1
  connections:
  -/RConn1 -- Voltage Sensor/RConn2
  +/RConn1 -- Voltage Sensor/LConn1
  Voltage Sensor/RConn1 -- PS-Simulink/LConn1

== system engv2_Simscape_test_no_graphs/Voltage Sensor Resistor 2 ==
  PS-Simulink : nesl_utility/PS-Simulink Converter  PhysicalDomain=network_engine_domain  SubClassName=ps_output  LeftPortType=input  RightPortType=output  PseudoPeriodic=off  Frequencies=[]  Unit=V  AffineConversion=off
  Voltage Sensor : fl_lib/Electrical/Electrical Sensors/Voltage Sensor
  + : PMIOPort  Port=1  Side=Left
  - : PMIOPort  Port=2  Side=Left
  v : Outport
  wires:
  PS-Simulink/1 -> v/1
  connections:
  -/RConn1 -- Voltage Sensor/RConn2
  +/RConn1 -- Voltage Sensor/LConn1
  Voltage Sensor/RConn1 -- PS-Simulink/LConn1

== system engv2_Simscape_test_no_graphs/Voltage Sensor Resistor 3 ==
  PS-Simulink : nesl_utility/PS-Simulink Converter  PhysicalDomain=network_engine_domain  SubClassName=ps_output  LeftPortType=input  RightPortType=output  PseudoPeriodic=off  Frequencies=[]  Unit=V  AffineConversion=off
  Voltage Sensor : fl_lib/Electrical/Electrical Sensors/Voltage Sensor
  + : PMIOPort  Port=1  Side=Left
  - : PMIOPort  Port=2  Side=Left
  v : Outport
  wires:
  PS-Simulink/1 -> v/1
  connections:
  -/RConn1 -- Voltage Sensor/RConn2
  +/RConn1 -- Voltage Sensor/LConn1
  Voltage Sensor/RConn1 -- PS-Simulink/LConn1

== system engv2_Simscape_test_no_graphs/Voltage Sensor Panel 1 ==
  PS-Simulink : nesl_utility/PS-Simulink Converter  PhysicalDomain=network_engine_domain  SubClassName=ps_output  LeftPortType=input  RightPortType=output  PseudoPeriodic=off  Frequencies=[]  Unit=V  AffineConversion=off
  Voltage Sensor : fl_lib/Electrical/Electrical Sensors/Voltage Sensor
  + : PMIOPort  Port=1  Side=Left
  - : PMIOPort  Port=2  Side=Left
  v : Outport
  wires:
  PS-Simulink/1 -> v/1
  connections:
  -/RConn1 -- Voltage Sensor/RConn2
  +/RConn1 -- Voltage Sensor/LConn1
  Voltage Sensor/RConn1 -- PS-Simulink/LConn1

== system engv2_Simscape_test_no_graphs/Voltage Sensor Panel 2 ==
  PS-Simulink : nesl_utility/PS-Simulink Converter  PhysicalDomain=network_engine_domain  SubClassName=ps_output  LeftPortType=input  RightPortType=output  PseudoPeriodic=off  Frequencies=[]  Unit=V  AffineConversion=off
  Voltage Sensor : fl_lib/Electrical/Electrical Sensors/Voltage Sensor
  + : PMIOPort  Port=1  Side=Left
  - : PMIOPort  Port=2  Side=Left
  v : Outport
  wires:
  PS-Simulink/1 -> v/1
  connections:
  -/RConn1 -- Voltage Sensor/RConn2
  +/RConn1 -- Voltage Sensor/LConn1
  Voltage Sensor/RConn1 -- PS-Simulink/LConn1

== system engv2_Simscape_test_no_graphs/Voltage Sensor Panel 3 ==
  PS-Simulink : nesl_utility/PS-Simulink Converter  PhysicalDomain=network_engine_domain  SubClassName=ps_output  LeftPortType=input  RightPortType=output  PseudoPeriodic=off  Frequencies=[]  Unit=V  AffineConversion=off
  Voltage Sensor : fl_lib/Electrical/Electrical Sensors/Voltage Sensor
  + : PMIOPort  Port=1  Side=Left
  - : PMIOPort  Port=2  Side=Left
  v : Outport
  wires:
  PS-Simulink/1 -> v/1
  connections:
  -/RConn1 -- Voltage Sensor/RConn2
  +/RConn1 -- Voltage Sensor/LConn1
  Voltage Sensor/RConn1 -- PS-Simulink/LConn1

== system engv2_Simscape_test_no_graphs/ Battery/Voltage Sensor (SL) ==
  PS-Simulink : nesl_utility/PS-Simulink Converter  PhysicalDomain=network_engine_domain  SubClassName=ps_output  LeftPortType=input  RightPortType=output  PseudoPeriodic=off  Frequencies=[]  Unit=V  AffineConversion=off
  Voltage Sensor : fl_lib/Electrical/Electrical Sensors/Voltage Sensor
  + : PMIOPort  Port=1  Side=Left
  - : PMIOPort  Port=2  Side=Left
  v : Outport
  wires:
  PS-Simulink/1 -> v/1
  connections:
  -/RConn1 -- Voltage Sensor/RConn2
  +/RConn1 -- Voltage Sensor/LConn1
  Voltage Sensor/RConn1 -- PS-Simulink/LConn1

== system engv2_Simscape_test_no_graphs/ Battery1/Voltage Sensor (SL) ==
  PS-Simulink : nesl_utility/PS-Simulink Converter  PhysicalDomain=network_engine_domain  SubClassName=ps_output  LeftPortType=input  RightPortType=output  PseudoPeriodic=off  Frequencies=[]  Unit=V  AffineConversion=off
  Voltage Sensor : fl_lib/Electrical/Electrical Sensors/Voltage Sensor
  + : PMIOPort  Port=1  Side=Left
  - : PMIOPort  Port=2  Side=Left
  v : Outport
  wires:
  PS-Simulink/1 -> v/1
  connections:
  -/RConn1 -- Voltage Sensor/RConn2
  +/RConn1 -- Voltage Sensor/LConn1
  Voltage Sensor/RConn1 -- PS-Simulink/LConn1

== system engv2_Simscape_test_no_graphs/Solar Panel 1/If Action Subsystem ==
  In1 : Inport
  In2 : Inport  Port=2
  Action Port : ActionPort  ActionType=then
  Out1 : Outport
  Out2 : Outport  Port=2
  wires:
  In1/1 -> Out1/1
  In2/1 -> Out2/1

== system engv2_Simscape_test_no_graphs/Solar Panel 1/If Action Subsystem1 ==
  In1 : Inport
  In2 : Inport  Port=2
  Action Port : ActionPort  ActionType=elseif
  Out1 : Outport
  Out2 : Outport  Port=2
  wires:
  In1/1 -> Out1/1
  In2/1 -> Out2/1

== system engv2_Simscape_test_no_graphs/Solar Panel 1/If Action Subsystem2 ==
  In1 : Inport
  In2 : Inport  Port=2
  Action Port : ActionPort  ActionType=else
  Out1 : Outport
  Out2 : Outport  Port=2
  wires:
  In1/1 -> Out1/1
  In2/1 -> Out2/1

== system engv2_Simscape_test_no_graphs/Solar Panel 2/If Action Subsystem ==
  In1 : Inport
  In2 : Inport  Port=2
  Action Port : ActionPort  ActionType=then
  Out1 : Outport
  Out2 : Outport  Port=2
  wires:
  In1/1 -> Out1/1
  In2/1 -> Out2/1

== system engv2_Simscape_test_no_graphs/Solar Panel 2/If Action Subsystem1 ==
  In1 : Inport
  In2 : Inport  Port=2
  Action Port : ActionPort  ActionType=elseif
  Out1 : Outport
  Out2 : Outport  Port=2
  wires:
  In1/1 -> Out1/1
  In2/1 -> Out2/1

== system engv2_Simscape_test_no_graphs/Solar Panel 2/If Action Subsystem2 ==
  In1 : Inport
  In2 : Inport  Port=2
  Action Port : ActionPort  ActionType=else
  Out1 : Outport
  Out2 : Outport  Port=2
  wires:
  In1/1 -> Out1/1
  In2/1 -> Out2/1

== system engv2_Simscape_test_no_graphs/Solar Panel 3/If Action Subsystem ==
  In1 : Inport
  In2 : Inport  Port=2
  Action Port : ActionPort  ActionType=then
  Out1 : Outport
  Out2 : Outport  Port=2
  wires:
  In1/1 -> Out1/1
  In2/1 -> Out2/1

== system engv2_Simscape_test_no_graphs/Solar Panel 3/If Action Subsystem1 ==
  In1 : Inport
  In2 : Inport  Port=2
  Action Port : ActionPort  ActionType=elseif
  Out1 : Outport
  Out2 : Outport  Port=2
  wires:
  In1/1 -> Out1/1
  In2/1 -> Out2/1

== system engv2_Simscape_test_no_graphs/Solar Panel 3/If Action Subsystem2 ==
  In1 : Inport
  In2 : Inport  Port=2
  Action Port : ActionPort  ActionType=else
  Out1 : Outport
  Out2 : Outport  Port=2
  wires:
  In1/1 -> Out1/1
  In2/1 -> Out2/1

== matlab function engv2_Simscape_test_no_graphs/MPPT1/MATLAB Function ==
  data: previous_voltage input; y output; previous_power input; voltage input; power input; bus_voltage input
function y = fcn(previous_voltage, previous_power, voltage, power, bus_voltage)

if power > previous_power
    if voltage > previous_voltage
        y = voltage - bus_voltage + 0.1;
    else
        y = voltage - bus_voltage - 0.1;
    end
else
    if voltage > previous_voltage
        y = voltage - bus_voltage - 0.1;
    else
        y = voltage - bus_voltage + 0.1;
    end
end

%{
if y > -2
    y = -4.2;
end
%}

== matlab function engv2_Simscape_test_no_graphs/MPPT/MATLAB Function ==
  data: previous_voltage input; y output; previous_power input; voltage input; power input; bus_voltage input
function y = fcn(previous_voltage, previous_power, voltage, power, bus_voltage)

if power > previous_power
    if voltage > previous_voltage
        y = voltage - bus_voltage + 0.1;
    else
        y = voltage - bus_voltage - 0.1;
    end
else
    if voltage > previous_voltage
        y = voltage - bus_voltage - 0.1;
    else
        y = voltage - bus_voltage + 0.1;
    end
end

%{
if y > -2
    y = -4.2;
end
%}

== matlab function engv2_Simscape_test_no_graphs/MPPT2/MATLAB Function ==
  data: previous_voltage input; y output; previous_power input; voltage input; power input; bus_voltage input
function y = fcn(previous_voltage, previous_power, voltage, power, bus_voltage)

if power > previous_power
    if voltage > previous_voltage
        y = voltage - bus_voltage + 0.1;
    else
        y = voltage - bus_voltage - 0.1;
    end
else
    if voltage > previous_voltage
        y = voltage - bus_voltage - 0.1;
    else
        y = voltage - bus_voltage + 0.1;
    end
end

%{
if y > -2
    y = -4.2;
end
%}
